simulink model "disturbance"  (R2022a)
settings: Solver=VariableStepAuto  StartTime=0.0  StopTime=100.0  RelTol=1e-3
undefined symbols (not defined in the file): fuzzy_triangle
libraries: fuzblock x1
settings Model: Creator=ark  LastModifiedBy=ark

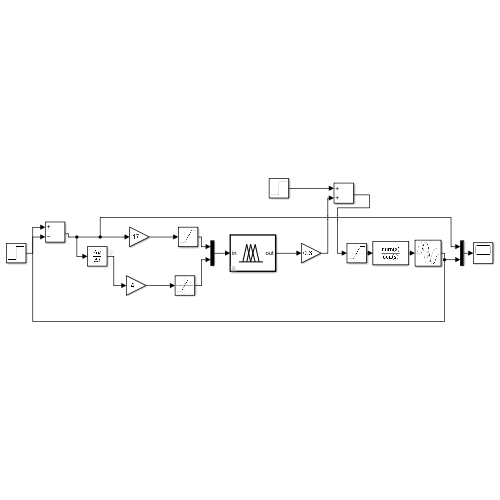
[thumbnail: Simulink's stored preview of the top-level diagram]
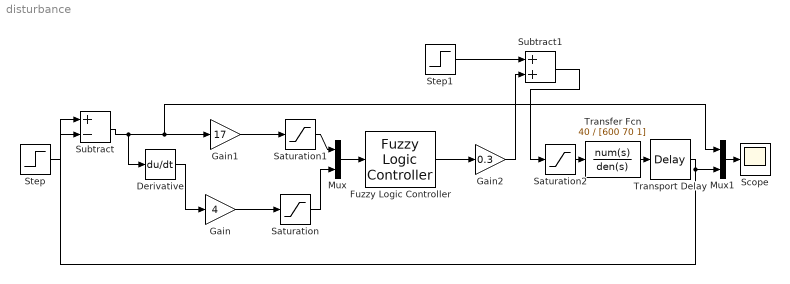
== system disturbance ==
  Derivative : Derivative
  Fuzzy Logic Controller : fuzblock/Fuzzy Logic  Controller  FIS=[fuzzy_triangle]  OutputSampleNumber=101  DataType=double  FuzzifiedInputs=off  RuleFiringStrengths=off  RuleOutputs=off  AggregatedOutputs=off  SimulateUsing=Interpreted execution  OutOfRangeInputValueMessage=warning  NoRuleFiredMessage=warning  EmptyOutputFuzzySetMessage=warning
  Gain : Gain  Gain=4
  Gain1 : Gain  Gain=17
  Gain2 : Gain  Gain=0.3
  Mux : Mux  Inputs=2
  Mux1 : Mux  Inputs=2
  Saturation : Saturate  UpperLimit=6  LowerLimit=-6
  Saturation1 : Saturate  UpperLimit=6  LowerLimit=-6
  Saturation2 : Saturate  UpperLimit=7  LowerLimit=-7
  Scope : Scope
  Step : Step  SampleTime=0
  Step1 : Step  SampleTime=0
  Subtract : Sum  Inputs=+-
  Subtract1 : Sum
  Transfer Fcn : TransferFcn  Numerator=40  Denominator=[600 70 1]
  Transport Delay : TransportDelay  DelayTime=2
  wires:
  Fuzzy Logic Controller/1 -> Gain2/1
  Gain1/1 -> Saturation1/1
  Saturation2/1 -> Transfer Fcn/1
  Subtract/1 -> Mux1/1, Gain1/1, Derivative/1
  Transfer Fcn/1 -> Transport Delay/1
  Gain/1 -> Saturation/1
  Transport Delay/1 -> Mux1/2, Subtract/2
  Gain2/1 -> Subtract1/2
  Derivative/1 -> Gain/1
  Step/1 -> Subtract/1
  Step1/1 -> Subtract1/1
  Subtract1/1 -> Saturation2/1
  Mux/1 -> Fuzzy Logic Controller/1
  Saturation1/1 -> Mux/1
  Saturation/1 -> Mux/2
  Mux1/1 -> Scope/1
